simulink model "demo"  (R2021b)
settings: Solver=VariableStepAuto  StartTime=0.0  StopTime=10  RelTol=1e-3
undefined symbols (not defined in the file or in its folder): xc7vx485tffg1157
libraries: hdlBasic x1736, vmcUtilities x1
(part 5 of 7)

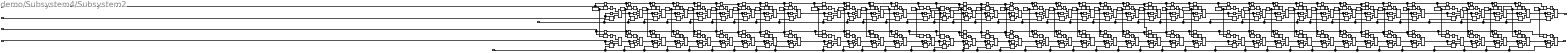
== system demo/Subsystem4/Subsystem2 ==
  note: 110
  note: 125
  note: 120
  note: 100
  note: 90
  In1 : Inport
  In2 : Inport  Port=2
  In3 : Inport  Port=3
  In4 : Inport  Port=4
  In5 : Inport  Port=5
  In6 : Inport  Port=6
  AddSub{102,104,113,138,140,164..171,184..190,192..193,195..200,205..207,209..211,236,238,249..250,252,254..258,261..269,271..280,282..291,293..299} (80 alike) : hdlBasic/AddSub  mode=Addition  use_carryin=off  use_carryout=off  en=off  latency=1  precision=User Defined  arith_type="Signed  (2's comp)"  n_bits=32  bin_pt=0  quantization=Truncate  overflow=Wrap  use_behavioral_HDL=off  hw_selection=Fabric  pipelined=off  XmcBlockStatus=1  maskContainerNames=tabcontainer1  block_type=addsub  block_config=sysgen:Addsub_config
  Delay{231..234,390..392,394,396..398,400,406..407,410..412,414,416..418,421,423,426..427,430..431,435,438,440,442..443,488,490..491,493..494,498..499,501..502,504..505,508..510,512..513,515..516,521..522,524..525,527,529,611..614,624..625,636..637,639..640,655..656,658..659,661..662,677..678,680..681,683..686,688,690..692,694,696..697,700..701,703..706,708,710..713,715,717,720..721,724..725,727,729,731..732,734,736..737,742..743,746..747,749..750,752..753,755,757,759..760,762..763,766,768,770..771,773..774,776..777,779,781..782,784..785,787..788,792..793,795..796,798..799,802..804,806..807,809..810,813,815..816,818..819,821,823} (160 alike) : hdlBasic/Delay  rst=off  en=off  latency=1  reg_retiming=off  XmcBlockStatus=1  maskContainerNames=group1  block_type=delay  block_config=sysgen:Delay_config
  Delay{395,399,405,408,415,420,424,428,432,436,441,444,489,492,496..497,500,503,507,511,514,518,520,523,526,530,635,638,657,660,679,682,689,693,695,699,702,709,714,718..719,722,726,730,735,738..739,741,744,748,751,754,758,761,764..765,769,772,775,780,783,786,790..791,794,797,801,805,808,812,814,817,820,824} (74 alike) : hdlBasic/Delay  rst=off  en=off  latency=2  reg_retiming=off  XmcBlockStatus=1  maskContainerNames=group1  block_type=delay  block_config=sysgen:Delay_config
  Mux{137..138,159..160,162..169,181..182,184..189,191..193,195..197,199..200,204..207,237..238,247..249,254..260,262..271,273..282,284..293,295..300} (80 alike) : hdlBasic/Mux  inputs=2  en=off  latency=1  precision=Full  arith_type=Unsigned  n_bits=16  bin_pt=14  quantization=Truncate  overflow=Wrap  XmcBlockStatus=1  maskContainerNames=tabcontainer1  block_type=mux  block_config=sysgen:Mux_config
  Relational{101,138..139,164..173,184,186..191,193..195,197..200,202..208,210,238..239,250,253,258..262,264..273,275..284,286..295,297..302} (80 alike) : hdlBasic/Relational  mode=a>=b  op_type=Bool  en=off  latency=1  XmcBlockStatus=1  maskContainerNames=tabcontainer1  block_type=relational  block_config=sysgen:Relational_config
  logi_b100 : hdlBasic/Constant  const=0.6129032258064516236473195931466761976480484008789062500  gui_display_data_type=Floating-point  arith_type=Floating-point  n_bits=8  bin_pt=8  preci_type=Double  exp_width=8  frac_width=24  explicit_period=on  period=1  XmcBlockStatus=1  maskContainerNames=tabcontainer1  block_type=constant  block_config=sysgen:Constant_config
  logi_b101 : hdlBasic/Constant  const=0.6290322580645161254508934689511079341173171997070312500  gui_display_data_type=Floating-point  arith_type=Floating-point  n_bits=8  bin_pt=8  preci_type=Double  exp_width=8  frac_width=24  explicit_period=on  period=1  XmcBlockStatus=1  maskContainerNames=tabcontainer1  block_type=constant  block_config=sysgen:Constant_config
  logi_b102 : hdlBasic/Constant  const=0.6451612903225806272544673447555396705865859985351562500  gui_display_data_type=Floating-point  arith_type=Floating-point  n_bits=8  bin_pt=8  preci_type=Double  exp_width=8  frac_width=24  explicit_period=on  period=1  XmcBlockStatus=1  maskContainerNames=tabcontainer1  block_type=constant  block_config=sysgen:Constant_config
  logi_b103 : hdlBasic/Constant  const=0.6612903225806451290580412205599714070558547973632812500  gui_display_data_type=Floating-point  arith_type=Floating-point  n_bits=8  bin_pt=8  preci_type=Double  exp_width=8  frac_width=24  explicit_period=on  period=1  XmcBlockStatus=1  maskContainerNames=tabcontainer1  block_type=constant  block_config=sysgen:Constant_config
  logi_b104 : hdlBasic/Constant  const=0.6774193548387096308616150963644031435251235961914062500  gui_display_data_type=Floating-point  arith_type=Floating-point  n_bits=8  bin_pt=8  preci_type=Double  exp_width=8  frac_width=24  explicit_period=on  period=1  XmcBlockStatus=1  maskContainerNames=tabcontainer1  block_type=constant  block_config=sysgen:Constant_config
  logi_b105 : hdlBasic/Constant  const=0.6935483870967741326651889721688348799943923950195312500  gui_display_data_type=Floating-point  arith_type=Floating-point  n_bits=8  bin_pt=8  preci_type=Double  exp_width=8  frac_width=24  explicit_period=on  period=1  XmcBlockStatus=1  maskContainerNames=tabcontainer1  block_type=constant  block_config=sysgen:Constant_config
  logi_b106 : hdlBasic/Constant  const=0.7096774193548387454910653104889206588268280029296875000  gui_display_data_type=Floating-point  arith_type=Floating-point  n_bits=8  bin_pt=8  preci_type=Double  exp_width=8  frac_width=24  explicit_period=on  period=1  XmcBlockStatus=1  maskContainerNames=tabcontainer1  block_type=constant  block_config=sysgen:Constant_config
  logi_b107 : hdlBasic/Constant  const=0.7258064516129032472946391862933523952960968017578125000  gui_display_data_type=Floating-point  arith_type=Floating-point  n_bits=8  bin_pt=8  preci_type=Double  exp_width=8  frac_width=24  explicit_period=on  period=1  XmcBlockStatus=1  maskContainerNames=tabcontainer1  block_type=constant  block_config=sysgen:Constant_config
  logi_b108 : hdlBasic/Constant  const=0.7419354838709677490982130620977841317653656005859375000  gui_display_data_type=Floating-point  arith_type=Floating-point  n_bits=8  bin_pt=8  preci_type=Double  exp_width=8  frac_width=24  explicit_period=on  period=1  XmcBlockStatus=1  maskContainerNames=tabcontainer1  block_type=constant  block_config=sysgen:Constant_config
  logi_b109 : hdlBasic/Constant  const=0.7580645161290322509017869379022158682346343994140625000  gui_display_data_type=Floating-point  arith_type=Floating-point  n_bits=8  bin_pt=8  preci_type=Double  exp_width=8  frac_width=24  explicit_period=on  period=1  XmcBlockStatus=1  maskContainerNames=tabcontainer1  block_type=constant  block_config=sysgen:Constant_config
  logi_b110 : hdlBasic/Constant  const=0.7741935483870967527053608137066476047039031982421875000  gui_display_data_type=Floating-point  arith_type=Floating-point  n_bits=8  bin_pt=8  preci_type=Double  exp_width=8  frac_width=24  explicit_period=on  period=1  XmcBlockStatus=1  maskContainerNames=tabcontainer1  block_type=constant  block_config=sysgen:Constant_config
  logi_b111 : hdlBasic/Constant  const=0.7903225806451612545089346895110793411731719970703125000  gui_display_data_type=Floating-point  arith_type=Floating-point  n_bits=8  bin_pt=8  preci_type=Double  exp_width=8  frac_width=24  explicit_period=on  period=1  XmcBlockStatus=1  maskContainerNames=tabcontainer1  block_type=constant  block_config=sysgen:Constant_config
  logi_b112 : hdlBasic/Constant  const=0.8064516129032257563125085653155110776424407958984375000  gui_display_data_type=Floating-point  arith_type=Floating-point  n_bits=8  bin_pt=8  preci_type=Double  exp_width=8  frac_width=24  explicit_period=on  period=1  XmcBlockStatus=1  maskContainerNames=tabcontainer1  block_type=constant  block_config=sysgen:Constant_config
  logi_b113 : hdlBasic/Constant  const=0.8225806451612902581160824411199428141117095947265625000  gui_display_data_type=Floating-point  arith_type=Floating-point  n_bits=8  bin_pt=8  preci_type=Double  exp_width=8  frac_width=24  explicit_period=on  period=1  XmcBlockStatus=1  maskContainerNames=tabcontainer1  block_type=constant  block_config=sysgen:Constant_config
  logi_b114 : hdlBasic/Constant  const=0.8387096774193547599196563169243745505809783935546875000  gui_display_data_type=Floating-point  arith_type=Floating-point  n_bits=8  bin_pt=8  preci_type=Double  exp_width=8  frac_width=24  explicit_period=on  period=1  XmcBlockStatus=1  maskContainerNames=tabcontainer1  block_type=constant  block_config=sysgen:Constant_config
  logi_b115 : hdlBasic/Constant  const=0.8548387096774193727455326552444603294134140014648437500  gui_display_data_type=Floating-point  arith_type=Floating-point  n_bits=8  bin_pt=8  preci_type=Double  exp_width=8  frac_width=24  explicit_period=on  period=1  XmcBlockStatus=1  maskContainerNames=tabcontainer1  block_type=constant  block_config=sysgen:Constant_config
  logi_b116 : hdlBasic/Constant  const=0.8709677419354838745491065310488920658826828002929687500  gui_display_data_type=Floating-point  arith_type=Floating-point  n_bits=8  bin_pt=8  preci_type=Double  exp_width=8  frac_width=24  explicit_period=on  period=1  XmcBlockStatus=1  maskContainerNames=tabcontainer1  block_type=constant  block_config=sysgen:Constant_config
  logi_b117 : hdlBasic/Constant  const=0.8870967741935483763526804068533238023519515991210937500  gui_display_data_type=Floating-point  arith_type=Floating-point  n_bits=8  bin_pt=8  preci_type=Double  exp_width=8  frac_width=24  explicit_period=on  period=1  XmcBlockStatus=1  maskContainerNames=tabcontainer1  block_type=constant  block_config=sysgen:Constant_config
  logi_b118 : hdlBasic/Constant  const=0.9032258064516128781562542826577555388212203979492187500  gui_display_data_type=Floating-point  arith_type=Floating-point  n_bits=8  bin_pt=8  preci_type=Double  exp_width=8  frac_width=24  explicit_period=on  period=1  XmcBlockStatus=1  maskContainerNames=tabcontainer1  block_type=constant  block_config=sysgen:Constant_config
  logi_b119 : hdlBasic/Constant  const=0.9193548387096773799598281584621872752904891967773437500  gui_display_data_type=Floating-point  arith_type=Floating-point  n_bits=8  bin_pt=8  preci_type=Double  exp_width=8  frac_width=24  explicit_period=on  period=1  XmcBlockStatus=1  maskContainerNames=tabcontainer1  block_type=constant  block_config=sysgen:Constant_config
  logi_b120 : hdlBasic/Constant  const=0.9354838709677418817634020342666190117597579956054687500  gui_display_data_type=Floating-point  arith_type=Floating-point  n_bits=8  bin_pt=8  preci_type=Double  exp_width=8  frac_width=24  explicit_period=on  period=1  XmcBlockStatus=1  maskContainerNames=tabcontainer1  block_type=constant  block_config=sysgen:Constant_config
  logi_b121 : hdlBasic/Constant  const=0.9516129032258063835669759100710507482290267944335937500  gui_display_data_type=Floating-point  arith_type=Floating-point  n_bits=8  bin_pt=8  preci_type=Double  exp_width=8  frac_width=24  explicit_period=on  period=1  XmcBlockStatus=1  maskContainerNames=tabcontainer1  block_type=constant  block_config=sysgen:Constant_config
  logi_b122 : hdlBasic/Constant  const=0.9677419354838709963928522483911365270614624023437500000  gui_display_data_type=Floating-point  arith_type=Floating-point  n_bits=8  bin_pt=8  preci_type=Double  exp_width=8  frac_width=24  explicit_period=on  period=1  XmcBlockStatus=1  maskContainerNames=tabcontainer1  block_type=constant  block_config=sysgen:Constant_config
  logi_b123 : hdlBasic/Constant  const=0.9838709677419354981964261241955682635307312011718750000  gui_display_data_type=Floating-point  arith_type=Floating-point  n_bits=8  bin_pt=8  preci_type=Double  exp_width=8  frac_width=24  explicit_period=on  period=1  XmcBlockStatus=1  maskContainerNames=tabcontainer1  block_type=constant  block_config=sysgen:Constant_config
  logi_b124 : hdlBasic/Constant  const=1.0000000000000000000000000000000000000000000000000000000  gui_display_data_type=Floating-point  arith_type=Floating-point  n_bits=8  bin_pt=8  preci_type=Double  exp_width=8  frac_width=24  explicit_period=on  period=1  XmcBlockStatus=1  maskContainerNames=tabcontainer1  block_type=constant  block_config=sysgen:Constant_config
  logi_b85 : hdlBasic/Constant  const=0.3709677419354838745491065310488920658826828002929687500  gui_display_data_type=Floating-point  arith_type=Floating-point  n_bits=8  bin_pt=8  preci_type=Double  exp_width=8  frac_width=24  explicit_period=on  period=1  XmcBlockStatus=1  maskContainerNames=tabcontainer1  block_type=constant  block_config=sysgen:Constant_config
  logi_b86 : hdlBasic/Constant  const=0.3870967741935483763526804068533238023519515991210937500  gui_display_data_type=Floating-point  arith_type=Floating-point  n_bits=8  bin_pt=8  preci_type=Double  exp_width=8  frac_width=24  explicit_period=on  period=1  XmcBlockStatus=1  maskContainerNames=tabcontainer1  block_type=constant  block_config=sysgen:Constant_config
  logi_b87 : hdlBasic/Constant  const=0.4032258064516128781562542826577555388212203979492187500  gui_display_data_type=Floating-point  arith_type=Floating-point  n_bits=8  bin_pt=8  preci_type=Double  exp_width=8  frac_width=24  explicit_period=on  period=1  XmcBlockStatus=1  maskContainerNames=tabcontainer1  block_type=constant  block_config=sysgen:Constant_config
  logi_b88 : hdlBasic/Constant  const=0.4193548387096773799598281584621872752904891967773437500  gui_display_data_type=Floating-point  arith_type=Floating-point  n_bits=8  bin_pt=8  preci_type=Double  exp_width=8  frac_width=24  explicit_period=on  period=1  XmcBlockStatus=1  maskContainerNames=tabcontainer1  block_type=constant  block_config=sysgen:Constant_config
  logi_b89 : hdlBasic/Constant  const=0.4354838709677419372745532655244460329413414001464843750  gui_display_data_type=Floating-point  arith_type=Floating-point  n_bits=8  bin_pt=8  preci_type=Double  exp_width=8  frac_width=24  explicit_period=on  period=1  XmcBlockStatus=1  maskContainerNames=tabcontainer1  block_type=constant  block_config=sysgen:Constant_config
  logi_b90 : hdlBasic/Constant  const=0.4516129032258064390781271413288777694106101989746093750  gui_display_data_type=Floating-point  arith_type=Floating-point  n_bits=8  bin_pt=8  preci_type=Double  exp_width=8  frac_width=24  explicit_period=on  period=1  XmcBlockStatus=1  maskContainerNames=tabcontainer1  block_type=constant  block_config=sysgen:Constant_config
  logi_b91 : hdlBasic/Constant  const=0.4677419354838709408817010171333095058798789978027343750  gui_display_data_type=Floating-point  arith_type=Floating-point  n_bits=8  bin_pt=8  preci_type=Double  exp_width=8  frac_width=24  explicit_period=on  period=1  XmcBlockStatus=1  maskContainerNames=tabcontainer1  block_type=constant  block_config=sysgen:Constant_config
  logi_b92 : hdlBasic/Constant  const=0.4838709677419354981964261241955682635307312011718750000  gui_display_data_type=Floating-point  arith_type=Floating-point  n_bits=8  bin_pt=8  preci_type=Double  exp_width=8  frac_width=24  explicit_period=on  period=1  XmcBlockStatus=1  maskContainerNames=tabcontainer1  block_type=constant  block_config=sysgen:Constant_config
  logi_b93 : hdlBasic/Constant  const=0.5000000000000000000000000000000000000000000000000000000  gui_display_data_type=Floating-point  arith_type=Floating-point  n_bits=8  bin_pt=8  preci_type=Double  exp_width=8  frac_width=24  explicit_period=on  period=1  XmcBlockStatus=1  maskContainerNames=tabcontainer1  block_type=constant  block_config=sysgen:Constant_config
  logi_b94 : hdlBasic/Constant  const=0.5161290322580645018035738758044317364692687988281250000  gui_display_data_type=Floating-point  arith_type=Floating-point  n_bits=8  bin_pt=8  preci_type=Double  exp_width=8  frac_width=24  explicit_period=on  period=1  XmcBlockStatus=1  maskContainerNames=tabcontainer1  block_type=constant  block_config=sysgen:Constant_config
  logi_b95 : hdlBasic/Constant  const=0.5322580645161290036071477516088634729385375976562500000  gui_display_data_type=Floating-point  arith_type=Floating-point  n_bits=8  bin_pt=8  preci_type=Double  exp_width=8  frac_width=24  explicit_period=on  period=1  XmcBlockStatus=1  maskContainerNames=tabcontainer1  block_type=constant  block_config=sysgen:Constant_config
  logi_b96 : hdlBasic/Constant  const=0.5483870967741935054107216274132952094078063964843750000  gui_display_data_type=Floating-point  arith_type=Floating-point  n_bits=8  bin_pt=8  preci_type=Double  exp_width=8  frac_width=24  explicit_period=on  period=1  XmcBlockStatus=1  maskContainerNames=tabcontainer1  block_type=constant  block_config=sysgen:Constant_config
  logi_b97 : hdlBasic/Constant  const=0.5645161290322580072142955032177269458770751953125000000  gui_display_data_type=Floating-point  arith_type=Floating-point  n_bits=8  bin_pt=8  preci_type=Double  exp_width=8  frac_width=24  explicit_period=on  period=1  XmcBlockStatus=1  maskContainerNames=tabcontainer1  block_type=constant  block_config=sysgen:Constant_config
  logi_b98 : hdlBasic/Constant  const=0.5806451612903225090178693790221586823463439941406250000  gui_display_data_type=Floating-point  arith_type=Floating-point  n_bits=8  bin_pt=8  preci_type=Double  exp_width=8  frac_width=24  explicit_period=on  period=1  XmcBlockStatus=1  maskContainerNames=tabcontainer1  block_type=constant  block_config=sysgen:Constant_config
  logi_b99 : hdlBasic/Constant  const=0.5967741935483871218437457173422444611787796020507812500  gui_display_data_type=Floating-point  arith_type=Floating-point  n_bits=8  bin_pt=8  preci_type=Double  exp_width=8  frac_width=24  explicit_period=on  period=1  XmcBlockStatus=1  maskContainerNames=tabcontainer1  block_type=constant  block_config=sysgen:Constant_config
  Out1 : Outport
  Out2 : Outport  Port=2
  wires:
  Delay683/1 -> Mux270/2
  Relational189/1 -> Delay504/1
  Mux292/1 -> Delay712/1, AddSub207/1
  AddSub256/1 -> Mux256/3
  AddSub295/1 -> Mux293/3
  Delay749/1 -> Mux205/1
  Relational168/1 -> Delay515/1
  Delay703/1 -> Mux280/1
  Delay406/1 -> Mux192/1
  Delay788/1 -> Mux285/2
  AddSub288/1 -> Mux289/3
  AddSub261/1 -> Mux270/3
  Delay704/1 -> Mux291/1
  Delay776/1 -> Mux278/1
  Delay795/1 -> Mux287/1
  Delay659/1 -> Mux255/2
  Mux184/1 -> AddSub185/1, Delay494/1
  Delay411/1 -> Mux191/2
  Delay763/1 -> Mux274/2
  Relational286/1 -> Delay787/1
  Delay658/1 -> Mux255/1
  Delay715/1 -> Mux263/1
  Delay773/1 -> Mux277/1
  Relational203/1 -> Delay655/1
  AddSub271/1 -> Mux280/3
  AddSub297/1 -> Mux296/3
  Delay414/1 -> Mux193/2
  logi_b112/1 -> Relational266/2, Relational272/2
  Relational190/1 -> Delay508/1
  Delay747/1 -> Mux204/2
  Delay508/1 -> Mux189/1
  In5/1 -> Delay394/1, AddSub166/1
  Delay799/1 -> Mux288/2
  AddSub252/1 -> Mux249/3
  Delay781/1 -> Mux271/1
  Delay611/1 -> Mux238/1
  AddSub188/1 -> Mux187/3
  Delay416/1 -> Mux195/1
  Delay779/1 -> Mux279/2
  Delay417/1 -> Mux159/1
  AddSub284/1 -> Mux282/3
  AddSub291/1 -> Mux292/3
  AddSub254/1 -> Mux254/3
  Mux258/1 -> Delay683/1, AddSub261/1
  Relational194/1 -> Delay417/1
  Delay391/1 -> Mux182/2
  Delay656/1 -> Mux254/2
  AddSub192/1 -> Mux191/3
  Relational264/1 -> Delay691/1
  Mux204/1 -> AddSub206/1, Delay750/1
  Delay766/1 -> Mux275/1
  Delay770/1 -> Mux276/1
  Delay686/1 -> Mux264/1
  Delay488/1 -> Mux162/2
  Delay516/1 -> Mux167/2
  Delay821/1 -> Mux281/1
  AddSub280/1 -> Mux279/3
  Relational273/1 -> Delay684/1
  logi_b115/1 -> Relational269/2, Relational287/2
  Mux282/1 -> AddSub290/1, Delay705/1
  Delay423/1 -> Mux163/2
  Mux191/1 -> Delay414/1, AddSub197/1
  Delay612/1 -> Mux238/2
  AddSub293/1 -> Mux263/3
  Relational277/1 -> Delay759/1
  AddSub264/1 -> Mux264/3
  AddSub299/1 -> Mux204/3
  Delay427/1 -> Mux199/2
  Relational207/1 -> Delay746/1
  AddSub211/1 -> Mux260/3
  Mux195/1 -> AddSub199/1, Delay440/1
  AddSub282/1 -> Mux281/3
  Delay420/1 -> Delay424/1, Relational200/1
  Mux206/1 -> AddSub280/1, Delay779/1
  Delay737/1 -> Mux297/2
  Delay524/1 -> Mux169/1
  Delay233/1 -> Mux137/1
  Relational272/1 -> Delay694/1
  Mux289/1 -> AddSub291/1, Delay701/1
  AddSub168/1 -> Mux166/3
  AddSub209/1 -> Mux206/3
  Relational276/1 -> Delay781/1
  Delay412/1 -> Mux193/1
  logi_b86/1 -> Relational166/2, Relational172/2
  Delay719/1 -> Relational301/1, Delay739/1
  Delay814/1 -> Delay817/1, Relational270/1
  Mux159/1 -> AddSub195/1, Delay423/1
  AddSub196/1 -> Mux199/3
  Delay808/1 -> Relational268/1, Delay812/1
  Relational265/1 -> Delay686/1
  AddSub294/1 -> Mux299/3
  Delay752/1 -> Mux206/1
  Delay736/1 -> Mux297/1
  AddSub285/1 -> Mux286/3
  Relational238/1 -> Delay611/1
  AddSub164/1 -> Mux162/3
  Delay807/1 -> Mux266/2
  Relational268/1 -> Delay809/1
  Delay694/1 -> Mux262/1
  Relational199/1 -> Delay442/1
  Delay706/1 -> Mux293/1
  AddSub165/1 -> Mux184/3
  logi_b92/1 -> Relational173/2, Relational190/2
  Delay771/1 -> Mux276/2
  AddSub275/1 -> Mux275/3
  Delay762/1 -> Mux274/1
  Relational291/1 -> Delay704/1
  Relational253/1 -> Delay624/1
  Delay692/1 -> Mux260/2
  Delay515/1 -> Mux167/1
  Delay662/1 -> Mux256/2
  Delay769/1 -> Delay772/1, Relational281/1
  Delay407/1 -> Mux192/2
  logi_b108/1 -> Relational281/2, Relational208/2
  Delay430/1 -> Mux200/1
  Delay625/1 -> Mux249/2
  AddSub266/1 -> Mux266/3
  Delay504/1 -> Mux188/1
  Relational283/1 -> Delay776/1
  Mux279/1 -> Delay692/1, AddSub211/1
  Mux197/1 -> AddSub138/1, Delay234/1
  Relational300/1 -> Delay715/1
  Relational169/1 -> Delay521/1
  Delay513/1 -> Mux166/2
  AddSub166/1 -> Mux164/3
  Relational275/1 -> Delay755/1
  Mux207/1 -> Delay688/1, AddSub264/1
  Delay746/1 -> Mux204/1
  Delay496/1 -> Delay497/1, Relational187/1
  Mux168/1 -> AddSub171/1, Delay525/1
  Relational164/1 -> Delay397/1
  Delay682/1 -> Relational260/1, Delay638/1
  AddSub186/1 -> Mux182/3
  Relational287/1 -> Delay792/1
  logi_b110/1 -> Relational262/2, Relational275/2
  Mux271/1 -> AddSub273/1, Delay760/1
  Delay697/1 -> Mux207/2
  Delay491/1 -> Mux184/2
  logi_b91/1 -> Relational171/2, Relational189/2
  Delay444/1 -> Relational204/1, Relational250/1, Delay679/1, Relational139/1
  Delay442/1 -> Mux197/1
  Relational171/1 -> Delay527/1
  Mux265/1 -> AddSub266/1, Delay807/1
  Delay636/1 -> Mux258/1
  Relational259/1 -> Delay661/1
  Delay695/1 -> Relational292/1, Delay719/1
  AddSub283/1 -> Mux285/3
  Delay640/1 -> Mux257/2
  Delay806/1 -> Mux266/1
  Delay505/1 -> Mux188/2
  Delay415/1 -> Delay436/1, Relational197/1
  Delay500/1 -> Delay503/1, Relational189/1
  Mux286/1 -> AddSub286/1, Delay796/1
  Relational262/1 -> Delay696/1
  logi_b114/1 -> Relational268/2, Relational286/2
  Mux238/1 -> Out1/1
  Delay754/1 -> Relational264/1, Delay693/1
  Relational282/1 -> Delay813/1
  logi_b96/1 -> Relational198/2, Relational202/2
  Delay724/1 -> Mux300/1
  Delay614/1 -> Mux237/2
  Mux293/1 -> AddSub296/1, Delay729/1
  Delay755/1 -> Mux279/1
  Delay711/1 -> Mux259/1
  Delay709/1 -> Delay730/1, Relational297/1
  Delay801/1 -> Relational293/1, Delay699/1
  AddSub249/1 -> Mux247/3
  Delay527/1 -> Mux181/1
  Relational284/1 -> Delay784/1
  Delay734/1 -> Mux296/2
  Delay713/1 -> Mux280/2
  logi_b113/1 -> Relational267/2, Relational284/2
  AddSub205/1 -> Mux300/3
  AddSub140/1 -> Mux138/3
  Delay231/1 -> Mux138/1
  Delay726/1 -> Relational238/1
  logi_b111/1 -> Relational265/2, Relational264/2
  Mux193/1 -> AddSub198/1, Delay435/1
  Mux205/1 -> AddSub209/1, Delay753/1
  Relational271/1 -> Delay821/1
  AddSub276/1 -> Mux276/3
  logi_b109/1 -> Relational283/2, Relational210/2
  AddSub113/1 -> Mux160/3
  logi_b106/1 -> Relational279/2, Relational206/2
  Delay718/1 -> Relational302/1, Delay722/1
  Delay739/1 -> Delay741/1, Relational206/1
  Mux262/1 -> AddSub263/1, Delay785/1
  Mux181/1 -> AddSub186/1, Delay391/1
  Mux281/1 -> AddSub284/1, Delay685/1
  Delay399/1 -> Delay489/1, Relational172/1
  Delay803/1 -> Mux289/2
  AddSub189/1 -> Mux188/3
  Delay721/1 -> Mux299/2
  Delay699/1 -> Relational294/1, Delay714/1
  Delay395/1 -> Delay511/1, Relational166/1
  Delay731/1 -> Mux290/2
  Delay390/1 -> Mux182/1
  Mux164/1 -> AddSub167/1, Delay510/1
  Relational188/1 -> Delay501/1
  Delay819/1 -> Mux269/2
  AddSub138/1 -> Mux137/3
  Relational197/1 -> Delay416/1
  Delay701/1 -> Mux292/2
  Mux287/1 -> AddSub287/1, Delay799/1
  Delay408/1 -> Relational195/1, Delay415/1
  Mux256/1 -> AddSub258/1, Delay637/1
  Delay802/1 -> Mux289/1
  Delay523/1 -> Delay526/1, Relational171/1
  Mux188/1 -> AddSub190/1, Delay509/1
  Delay759/1 -> Mux273/1
  Delay410/1 -> Mux191/1
  Relational297/1 -> Delay710/1
  Delay660/1 -> Relational261/1, Delay635/1
  Delay435/1 -> Mux195/2
  Mux196/1 -> AddSub200/1, Delay443/1
  Mux277/1 -> AddSub279/1, Delay777/1
  logi_b95/1 -> Relational197/2, Relational200/2
  Delay400/1 -> Mux162/1
  AddSub197/1 -> Mux193/3
  Delay710/1 -> Mux295/1
  Mux162/1 -> AddSub165/1, Delay491/1
  Delay813/1 -> Mux270/1
  Delay730/1 -> Relational298/1, Delay735/1
  Mux297/1 -> AddSub236/1, Delay614/1
  Mux269/1 -> AddSub282/1, Delay823/1
  Delay529/1 -> Mux181/2
  Delay510/1 -> Mux165/2
  In1/1 -> Delay399/1, Relational164/1
  Delay748/1 -> Relational210/1, Delay751/1
  Delay440/1 -> Mux196/2
  logi_b122/1 -> Relational298/2, Relational302/2
  AddSub257/1 -> Mux257/3
  Delay783/1 -> Relational284/1, Delay786/1
  Delay398/1 -> Mux160/2
  AddSub184/1 -> Mux181/3
  Delay436/1 -> Relational198/1, Delay441/1
  Delay824/1 -> Relational291/1, Delay702/1
  Relational172/1 -> Delay400/1
  Delay493/1 -> Mux185/1
  Relational205/1 -> Delay724/1
  Delay761/1 -> Relational278/1, Delay764/1
  Delay232/1 -> Mux138/2
  Mux160/1 -> AddSub164/1, Delay488/1
  In3/1 -> AddSub165/2, AddSub185/2, AddSub187/2, AddSub188/2, AddSub189/2, AddSub104/2, AddSub196/2, AddSub238/2, AddSub205/2, AddSub294/2, AddSub293/2, AddSub207/2, AddSub291/2, AddSub288/2, AddSub287/2, AddSub286/2, AddSub285/2, AddSub283/2, AddSub263/2, AddSub262/2, AddSub211/2, AddSub280/2, AddSub209/2, AddSub206/2, AddSub299/2, AddSub289/2, AddSub278/2, AddSub271/2, AddSub261/2, AddSub258/2, AddSub256/2, AddSub255/2, AddSub254/2, AddSub140/2, AddSub102/2, AddSub195/2, AddSub193/2, AddSub190/2, AddSub164/2, AddSub113/2
  Delay443/1 -> Mux197/2
  Delay396/1 -> Mux165/1
  Mux166/1 -> AddSub169/1, Delay516/1
  Delay750/1 -> Mux205/2
  Delay431/1 -> Mux200/2
  Delay661/1 -> Mux256/1
  Delay637/1 -> Mux258/2
  AddSub193/1 -> Mux192/3
  Delay768/1 -> Mux275/2
  Relational289/1 -> Delay798/1
  Delay705/1 -> Mux291/2
  Delay426/1 -> Mux199/1
  Delay815/1 -> Mux268/1
  Mux268/1 -> AddSub269/1, Delay819/1
  logi_b88/1 -> Relational168/2, Relational186/2
  Delay518/1 -> Delay520/1, Relational169/1
  Delay689/1 -> Delay805/1, Relational266/1
  Mux298/1 -> AddSub299/1, Delay747/1
  Delay394/1 -> Mux164/2
  Mux259/1 -> AddSub293/1, Delay717/1
  Delay677/1 -> Mux247/1
  Delay520/1 -> Delay523/1, Relational170/1
  Relational292/1 -> Delay703/1
  Delay613/1 -> Mux237/1
  Mux276/1 -> AddSub277/1, Delay774/1
  Relational198/1 -> Delay438/1
  Delay785/1 -> Mux284/2
  Delay774/1 -> Mux277/2
  Delay432/1 -> Relational138/1, Relational203/1, Relational258/1, Delay657/1
  Delay717/1 -> Mux263/2
  AddSub170/1 -> Mux168/3
  logi_b124/1 -> Relational239/2, Relational238/2
  Delay691/1 -> Mux260/1
  Relational301/1 -> Delay727/1
  AddSub262/1 -> Mux262/3
  Delay525/1 -> Mux169/2
  Delay680/1 -> Mux248/1
  Delay688/1 -> Mux264/2
  Delay760/1 -> Mux273/2
  Mux189/1 -> AddSub193/1, Delay407/1
  Delay772/1 -> Relational283/1, Delay775/1
  Delay823/1 -> Mux281/2
  logi_b102/1 -> Relational260/2, Relational261/2
  Delay818/1 -> Mux269/1
  Delay720/1 -> Mux299/1
  Relational280/1 -> Delay770/1
  AddSub195/1 -> Mux163/3
  logi_b121/1 -> Relational297/2, Relational300/2
  Delay820/1 -> Relational273/1, Delay824/1
  Relational101/1 -> Delay430/1
  Delay744/1 -> Delay748/1, Relational208/1
  logi_b87/1 -> Relational167/2, Relational184/2
  Relational204/1 -> Delay677/1
  Delay512/1 -> Mux166/1
  Mux264/1 -> AddSub265/1, Delay804/1
  Delay702/1 -> Relational295/1, Delay709/1
  Delay775/1 -> Relational262/1, Delay780/1
  Relational184/1 -> Delay490/1
  Delay685/1 -> Mux282/2
  AddSub199/1 -> Mux196/3
  AddSub187/1 -> Mux186/3
  In6/1 -> AddSub166/2, AddSub197/2, AddSub236/2, AddSub298/2, AddSub297/2, AddSub296/2, AddSub295/2, AddSub290/2, AddSub284/2, AddSub282/2, AddSub269/2, AddSub268/2, AddSub267/2, AddSub266/2, AddSub265/2, AddSub264/2, AddSub210/2, AddSub279/2, AddSub277/2, AddSub276/2, AddSub275/2, AddSub274/2, AddSub273/2, AddSub272/2, AddSub257/2, AddSub252/2, AddSub250/2, AddSub249/2, AddSub138/2, AddSub200/2, AddSub199/2, AddSub198/2, AddSub192/2, AddSub186/2, AddSub184/2, AddSub171/2, AddSub170/2, AddSub169/2, AddSub168/2, AddSub167/2
  Relational250/1 -> Delay680/1
  Delay798/1 -> Mux288/1
  Relational170/1 -> Delay524/1
  Delay489/1 -> Relational184/1, Delay492/1
  logi_b120/1 -> Relational295/2, Relational294/2
  Delay708/1 -> Mux293/2
  Delay787/1 -> Mux285/1
  Mux288/1 -> AddSub288/1, Delay803/1
  Delay639/1 -> Mux257/1
  Delay725/1 -> Mux300/2
  Delay234/1 -> Mux137/2
  Mux280/1 -> AddSub278/1, Delay731/1
  Relational187/1 -> Delay498/1
  AddSub272/1 -> Mux271/3
  Delay498/1 -> Mux186/1
  Relational206/1 -> Delay742/1
  AddSub198/1 -> Mux195/3
  Mux165/1 -> AddSub168/1, Delay513/1
  Delay638/1 -> Delay758/1, Relational276/1
  Relational258/1 -> Delay658/1
  Mux237/1 -> Out2/1
  Delay511/1 -> Relational167/1, Delay514/1
  AddSub238/1 -> Mux238/3
  AddSub267/1 -> Mux267/3
  AddSub279/1 -> Mux278/3
  Delay405/1 -> Relational194/1, Delay420/1
  Delay742/1 -> Mux298/1
  Delay514/1 -> Relational168/1, Delay518/1
  Delay816/1 -> Mux268/2
  Relational138/1 -> Delay231/1
  logi_b89/1 -> Relational169/2, Relational187/2
  AddSub206/1 -> Mux205/3
  Mux167/1 -> AddSub170/1, Delay522/1
  Relational186/1 -> Delay493/1
  Delay507/1 -> Relational193/1, Delay405/1
  Delay804/1 -> Mux265/2
  Delay753/1 -> Mux206/2
  Mux186/1 -> AddSub188/1, Delay502/1
  Delay438/1 -> Mux196/1
  AddSub200/1 -> Mux197/3
  Mux247/1 -> AddSub250/1, Delay681/1
  Delay793/1 -> Mux286/2
  Delay758/1 -> Relational277/1, Delay761/1
  Relational139/1 -> Delay233/1
  Mux163/1 -> AddSub196/1, Delay427/1
  AddSub268/1 -> Mux268/3
  Mux137/1 -> AddSub249/1, Delay678/1
  Relational294/1 -> Delay711/1
  Mux169/1 -> AddSub184/1, Delay529/1
  Delay714/1 -> Delay718/1, Relational300/1
  Relational173/1 -> Delay390/1
  logi_b90/1 -> Relational170/2, Relational188/2
  Delay521/1 -> Mux168/1
  Delay797/1 -> Relational290/1, Delay801/1
  AddSub290/1 -> Mux291/3
  Relational208/1 -> Delay749/1
  AddSub250/1 -> Mux248/3
  AddSub190/1 -> Mux189/3
  Mux291/1 -> Delay708/1, AddSub295/1
  Relational278/1 -> Delay762/1
  AddSub102/1 -> Mux200/3
  AddSub287/1 -> Mux288/3
  Relational279/1 -> Delay766/1
  Mux285/1 -> AddSub285/1, Delay793/1
  logi_b85/1 -> Relational165/2, Relational164/2
  Mux274/1 -> AddSub275/1, Delay768/1
  Mux200/1 -> AddSub140/1, Delay232/1
  Delay812/1 -> Delay814/1, Relational269/1
  Mux278/1 -> AddSub210/1, Delay697/1
  Mux299/1 -> AddSub205/1, Delay725/1
  Mux257/1 -> Delay757/1, AddSub272/1
  Delay817/1 -> Delay820/1, Relational271/1
  Relational210/1 -> Delay752/1
  logi_b123/1 -> Relational299/2, Relational205/2
  logi_b104/1 -> Relational277/2, Relational292/2
  Delay494/1 -> Mux185/2
  Mux267/1 -> AddSub268/1, Delay816/1
  logi_b97/1 -> Relational199/2, Relational101/2
  Relational267/1 -> Delay806/1
  Relational288/1 -> Delay795/1
  Delay810/1 -> Mux267/2
  Mux275/1 -> AddSub276/1, Delay771/1
  Relational166/1 -> Delay396/1
  Mux273/1 -> AddSub274/1, Delay763/1
  logi_b105/1 -> Relational278/2, Relational301/2
  AddSub169/1 -> Mux167/3
  Delay792/1 -> Mux286/1
  AddSub273/1 -> Mux273/3
  Relational239/1 -> Delay613/1
  AddSub269/1 -> Mux269/3
  Delay729/1 -> Mux295/2
  Delay796/1 -> Mux287/2
  logi_b103/1 -> Relational276/2, Relational282/2
  Delay522/1 -> Mux168/2
  logi_b101/1 -> Relational253/2, Relational259/2
  logi_b116/1 -> Relational270/2, Relational288/2
  Delay712/1 -> Mux259/2
  Delay428/1 -> Relational101/1, Delay432/1
  AddSub277/1 -> Mux277/3
  Mux295/1 -> AddSub297/1, Delay734/1
  Delay700/1 -> Mux292/1
  Delay782/1 -> Mux262/2
  Mux192/1 -> Delay418/1, AddSub104/1
  In2/1 -> Delay398/1, AddSub113/1
  Delay679/1 -> Relational253/1, Delay682/1
  Delay392/1 -> Mux164/1
  Delay418/1 -> Mux159/2
  Mux300/1 -> AddSub238/1, Delay612/1
  Relational293/1 -> Delay700/1
  Delay497/1 -> Delay500/1, Relational188/1
  Relational302/1 -> Delay720/1
  Relational191/1 -> Delay410/1
  Relational195/1 -> Delay412/1
  Delay526/1 -> Relational173/1, Delay530/1
  Mux260/1 -> AddSub262/1, Delay782/1
  AddSub278/1 -> Mux290/3
  Delay421/1 -> Mux163/1
  Delay765/1 -> Delay769/1, Relational280/1
  AddSub258/1 -> Mux258/3
  In4/1 -> Relational165/1, Delay395/1
  AddSub236/1 -> Mux237/3
  Mux187/1 -> AddSub189/1, Delay505/1
  logi_b100/1 -> Relational250/2, Relational258/2
  Delay696/1 -> Mux207/1
  AddSub296/1 -> Mux295/3
  Mux284/1 -> AddSub283/1, Delay788/1
  Mux255/1 -> AddSub256/1, Delay662/1
  Delay501/1 -> Mux187/1
  Delay503/1 -> Relational190/1, Delay507/1
  Delay693/1 -> Delay783/1, Relational272/1
  Relational200/1 -> Delay421/1
  Mux296/1 -> AddSub298/1, Delay737/1
  Relational298/1 -> Delay732/1
  Delay790/1 -> Delay791/1, Relational287/1
  Delay684/1 -> Mux282/1
  logi_b99/1 -> Relational204/2, Relational203/2
  Delay624/1 -> Mux249/1
  Relational260/1 -> Delay639/1
  Delay490/1 -> Mux184/1
  Delay777/1 -> Mux278/2
  Delay757/1 -> Mux271/2
  Mux254/1 -> AddSub255/1, Delay659/1
  AddSub265/1 -> Mux265/3
  Mux266/1 -> AddSub267/1, Delay810/1
  Delay735/1 -> Relational299/1, Delay738/1
  Delay509/1 -> Mux189/2
  logi_b94/1 -> Relational195/2, Relational194/2
  AddSub104/1 -> Mux159/3
  logi_b118/1 -> Relational273/2, Relational290/2
  Relational202/1 -> Delay426/1
  Relational299/1 -> Delay736/1
  Delay727/1 -> Mux290/1
  Mux290/1 -> AddSub289/1, Delay743/1
  Relational281/1 -> Delay773/1
  AddSub167/1 -> Mux165/3
  Mux182/1 -> AddSub192/1, Delay411/1
  Mux138/1 -> AddSub254/1, Delay656/1
  Delay492/1 -> Relational186/1, Delay496/1
  Delay655/1 -> Mux254/1
  Delay441/1 -> Relational199/1, Delay444/1
  Delay530/1 -> Relational191/1, Delay408/1
  Delay764/1 -> Delay765/1, Relational279/1
  AddSub274/1 -> Mux274/3
  Delay786/1 -> Relational286/1, Delay790/1
  Relational270/1 -> Delay818/1
  AddSub286/1 -> Mux287/3
  Mux270/1 -> AddSub271/1, Delay713/1
  Delay741/1 -> Delay744/1, Relational207/1
  Mux263/1 -> AddSub294/1, Delay721/1
  Delay738/1 -> Relational239/1
  AddSub171/1 -> Mux169/3
  Mux185/1 -> AddSub187/1, Delay499/1
  Relational266/1 -> Delay690/1
  Delay809/1 -> Mux267/1
  logi_b107/1 -> Relational280/2, Relational207/2
  logi_b98/1 -> Relational139/2, Relational138/2
  Delay791/1 -> Delay794/1, Relational288/1
  Relational261/1 -> Delay636/1
  logi_b119/1 -> Relational291/2, Relational293/2
  Delay499/1 -> Mux186/2
  Delay784/1 -> Mux284/1
  AddSub289/1 -> Mux298/3
  Relational295/1 -> Delay706/1
  AddSub210/1 -> Mux207/3
  Relational193/1 -> Delay406/1
  Delay794/1 -> Delay797/1, Relational289/1
  Delay732/1 -> Mux296/1
  AddSub263/1 -> Mux284/3
  Delay751/1 -> Relational275/1, Delay754/1
  logi_b93/1 -> Relational191/2, Relational193/2
  Delay502/1 -> Mux187/2
  Delay743/1 -> Mux298/2
  Delay397/1 -> Mux160/1
  Relational269/1 -> Delay815/1
  Mux248/1 -> AddSub252/1, Delay625/1
  Mux249/1 -> AddSub257/1, Delay640/1
  Delay678/1 -> Mux247/2
  Delay635/1 -> Delay695/1, Relational282/1
  Delay805/1 -> Relational267/1, Delay808/1
  Relational167/1 -> Delay512/1
  Delay657/1 -> Relational259/1, Delay660/1
  Delay780/1 -> Relational265/1, Delay689/1
  Delay424/1 -> Relational202/1, Delay428/1
  Delay681/1 -> Mux248/2
  Delay690/1 -> Mux265/1
  AddSub298/1 -> Mux297/3
  Delay722/1 -> Relational205/1, Delay726/1
  Relational165/1 -> Delay392/1
  Mux199/1 -> AddSub102/1, Delay431/1
  Relational290/1 -> Delay802/1
  logi_b117/1 -> Relational271/2, Relational289/2
  AddSub185/1 -> Mux185/3
  AddSub207/1 -> Mux259/3
  AddSub255/1 -> Mux255/3

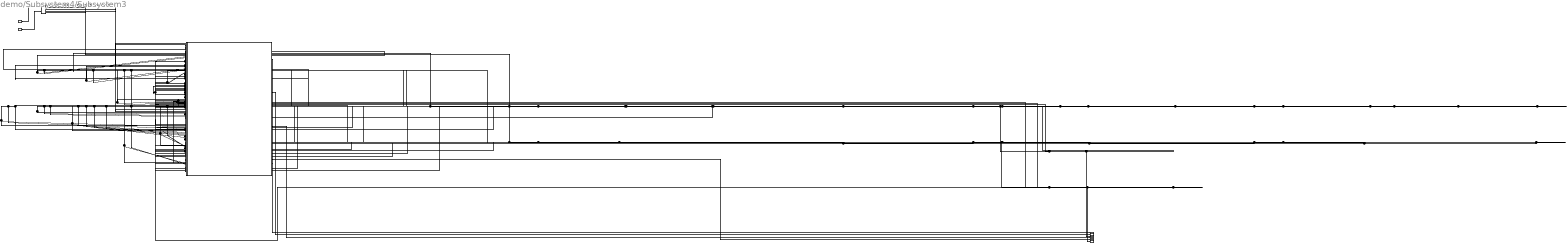
== system demo/Subsystem4/Subsystem3 ==
  In1 : Inport
  In2 : Inport  Port=2
  Subsystem : Subsystem
  Subsystem1 : Subsystem
  Out1 : Outport
  Out2 : Outport  Port=2
  Out3 : Outport  Port=3
  Out4 : Outport  Port=4
  Out5 : Outport  Port=5
  Out6 : Outport  Port=6
  wires:
  Subsystem/5(Out5) -> Subsystem1/53(In53)
  Subsystem1/1(Out1) -> Out1/1
  Subsystem/2(Out2) -> Subsystem1/2(In2)
  Subsystem1/2(Out2) -> Out2/1
  Subsystem/6(Out6) -> Subsystem1/64(In64), Subsystem1/65(In65), Subsystem1/66(In66), Subsystem1/67(In67), Subsystem1/62(In62), Subsystem1/78(In78), Subsystem1/79(In79), Subsystem1/80(In80), Subsystem1/81(In81), Subsystem1/97(In97), Subsystem1/96(In96), Subsystem1/98(In98), Subsystem1/95(In95), Subsystem1/90(In90), Subsystem1/85(In85), Subsystem1/83(In83), Subsystem1/82(In82), Subsystem1/84(In84), Subsystem1/102(In102), Subsystem1/100(In100), Subsystem1/99(In99), Subsystem1/101(In101), Subsystem1/91(In91), Subsystem1/88(In88), Subsystem1/87(In87), Subsystem1/86(In86), Subsystem1/77(In77), Subsystem1/75(In75), Subsystem1/74(In74), Subsystem1/76(In76), Subsystem1/63(In63), Out6/1, Subsystem1/61(In61), Subsystem1/59(In59), Subsystem1/58(In58), Subsystem1/60(In60), Subsystem1/89(In89), Subsystem1/92(In92), Subsystem1/93(In93), Subsystem1/94(In94), Subsystem1/68(In68), Subsystem1/69(In69), Subsystem1/70(In70), Subsystem1/71(In71), Subsystem1/72(In72), Subsystem1/73(In73), Subsystem1/54(In54), Subsystem1/55(In55), Subsystem1/56(In56), Subsystem1/57(In57)
  In2/1 -> Subsystem/2(In2)
  Subsystem1/4(Out4) -> Out5/1
  Subsystem/4(Out4) -> Subsystem1/52(In52)
  In1/1 -> Subsystem/1(In1)
  Subsystem/3(Out3) -> Subsystem1/29(In29), Subsystem1/30(In30), Subsystem1/49(In49), Subsystem1/48(In48), Subsystem1/42(In42), Subsystem1/37(In37), Subsystem1/36(In36), Subsystem1/35(In35), Subsystem1/24(In24), Subsystem1/31(In31), Subsystem1/32(In32), Subsystem1/51(In51), Subsystem1/50(In50), Subsystem1/43(In43), Subsystem1/40(In40), Subsystem1/39(In39), Subsystem1/38(In38), Subsystem1/28(In28), Subsystem1/26(In26), Subsystem1/25(In25), Subsystem1/27(In27), Out3/1, Subsystem1/4(In4), Subsystem1/5(In5), Subsystem1/13(In13), Subsystem1/14(In14), Subsystem1/16(In16), Subsystem1/22(In22), Subsystem1/23(In23), Subsystem1/33(In33), Subsystem1/34(In34), Subsystem1/41(In41), Subsystem1/44(In44), Subsystem1/45(In45), Subsystem1/46(In46), Subsystem1/47(In47), Subsystem1/19(In19), Subsystem1/20(In20), Subsystem1/21(In21), Subsystem1/9(In9), Subsystem1/8(In8), Subsystem1/3(In3), Subsystem1/10(In10), Subsystem1/11(In11), Subsystem1/12(In12), Subsystem1/15(In15), Subsystem1/18(In18), Subsystem1/17(In17), Subsystem1/6(In6), Subsystem1/7(In7)
  Subsystem1/3(Out3) -> Out4/1
  Subsystem/1(Out1) -> Subsystem1/1(In1)
